simulink model "simulazione_008_s"  (R2016b)
settings: Solver=ode4  StartTime=0.0  StopTime=t_sim  FixedStep=step  RelTol=1e-3
values from neighbouring files (symbols this model uses):
  final_theta = pi/3    (= 1.0471975512)    [simulazione_008_init.m]
  motion_time = 5    [simulazione_008_init.m]
  movement_lower_limit = -movement_upper_limit    [simulazione_008_init.m]
  movement_upper_limit = [2*pi; 2*pi; 2*pi; 2*pi; 2*pi; 2*pi]    [simulazione_008_init.m]
  p_init = direct_kinematic(q_init)    [simulazione_008_init.m]
  q_init = [pi/9; -pi/3; 2*pi/7; -pi/2; pi/4; pi/7]    [simulazione_008_init.m]
  radius = 0.4    [simulazione_008_init.m]
  velocity_lower_limit = -velocity_upper_limit    [simulazione_008_init.m]
  velocity_upper_limit = [2*pi/3; 2*pi/3; pi; pi; pi; pi]    [simulazione_008_init.m]
settings Model: Creator=IBM  LastModifiedBy=IBM

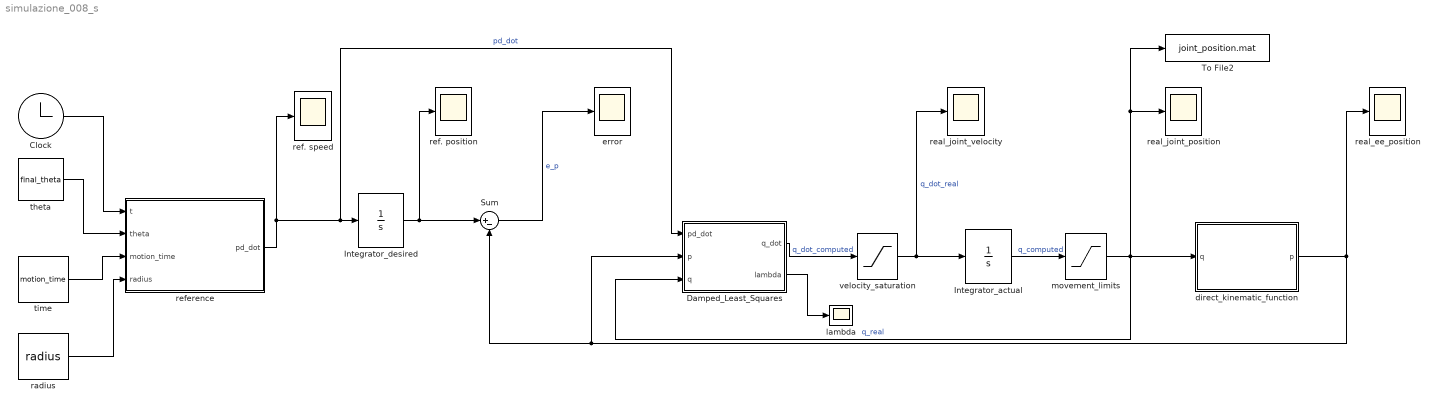
== system simulazione_008_s ==
  Clock : Clock
  Damped_Least_Squares : MATLAB Function  TreatAsAtomicUnit=on
  Integrator_actual : Integrator  InitialCondition=q_init
  Integrator_desired : Integrator  InitialCondition=p_init
  Sum : Sum  Inputs=|+-
  To File2 : ToFile  Filename=joint_position.mat  MatrixName=q
  direct_kinematic_function : MATLAB Function  TreatAsAtomicUnit=on
  error : Scope
  lambda : Scope
  movement_limits : Saturate  UpperLimit=movement_upper_limit  LowerLimit=movement_lower_limit
  radius : Constant  Value=radius
  real_ee_position : Scope
  real_joint_position : Scope
  real_joint_velocity : Scope
  ref. position : Scope
  ref. speed : Scope
  reference : MATLAB Function  TreatAsAtomicUnit=on
  theta : Constant  Value=final_theta
  time : Constant  Value=motion_time
  velocity_saturation : Saturate  UpperLimit=velocity_upper_limit  LowerLimit=velocity_lower_limit
  wires:
  Clock/1 -> reference/1(t)
  Integrator_desired/1 -> ref. position/1, Sum/1
  Sum/1 -> error/1  "e_p"
  direct_kinematic_function/1(p) -> real_ee_position/1, Damped_Least_Squares/2(p), Sum/2
  theta/1 -> reference/2(theta)
  reference/1(pd_dot) -> ref. speed/1, Damped_Least_Squares/1(pd_dot), Integrator_desired/1  "pd_dot"
  time/1 -> reference/3(motion_time)
  radius/1 -> reference/4(radius)
  Integrator_actual/1 -> movement_limits/1  "q_computed"
  movement_limits/1 -> Damped_Least_Squares/3(q), To File2/1, real_joint_position/1, direct_kinematic_function/1(q)  "q_real"
  Damped_Least_Squares/1(q_dot) -> velocity_saturation/1  "q_dot_computed"
  velocity_saturation/1 -> real_joint_velocity/1, Integrator_actual/1  "q_dot_real"
  Damped_Least_Squares/2(lambda) -> lambda/1

== matlab function simulazione_008_s/Damped_Least_Squares ==
  data: pd_dot input; p input; q_dot output; q input; lambda output
function [q_dot, lambda] = dls(pd_dot, p, q)

    Jg = geometric_jacobian(q);
    Ja = analytic_jacobian(Jg, p);
    
    s = svd(Ja);
    sigma_th = 1/pi;
    sigma = s(6);
    lambda_max = 0.00008;
    
    if sigma >= sigma_th 
        lambda = 0; 
    else
        lambda = lambda_max - lambda_max * sigma / sigma_th;
    end
    
    q_dot = transpose(Ja) * inv(Ja * transpose(Ja) + lambda * eye(6)) * pd_dot;
    
end

== matlab function simulazione_008_s/reference ==
  data: t input; theta input; pd_dot output; motion_time input; radius input
function pd_dot = reference(t, theta, motion_time, radius)

    pd_dot = rotational_reference(t, theta, motion_time, radius);
    
end

== matlab function simulazione_008_s/direct_kinematic_function ==
  data: q input; p output
function p = dkf(q)

    p = direct_kinematic(q);
